simulink model "TD"  (R2020a)
settings: Solver=VariableStepAuto  StartTime=0.0  StopTime=0.05  RelTol=1e-3
undefined symbols (not defined in the file or in its folder): R1, R2
libraries: powerlib x7
settings Model: Creator=eduh_  LastModifiedBy=eduh_

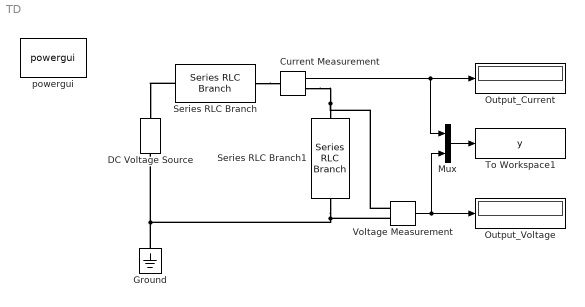
== system TD ==
  Current Measurement : powerlib/Measurements/Current Measurement  PhasorSimulation=off  OutputType=Complex  PSBequivalent=0
  DC Voltage Source : powerlib/Electrical Sources/DC Voltage Source  Amplitude=20  Measurements=None
  Ground : powerlib/Elements/Ground  LConnTagsString=a
  Mux : Mux  Inputs=2
  Output_Current : Display
      settings: Decimation=5
  Output_Voltage : Display
      settings: Decimation=5
  Series RLC Branch : powerlib/Elements/Series RLC Branch  LConnTagsString=__new0  RConnTagsString=__new0  BranchType=R  Resistance=R1  Inductance=0  SetiL0=off  InitialCurrent=0  Capacitance=0  Setx0=off  InitialVoltage=0  Measurements=None
  Series RLC Branch1 : powerlib/Elements/Series RLC Branch  LConnTagsString=__new0  RConnTagsString=__new0  BranchType=R  Resistance=R2  Inductance=0  SetiL0=off  InitialCurrent=0  Capacitance=0  Setx0=off  InitialVoltage=0  Measurements=None
  To Workspace1 : ToWorkspace  VariableName=y  SampleTime=1
      settings: MaxDataPoints=1  Save2DSignal=2-D array (concatenate along first dimension)
  Voltage Measurement : powerlib/Measurements/Voltage Measurement  PhasorSimulation=off  OutputType=Complex  PSBequivalent=0
  powergui : powerlib/powergui  Priority=1  SimulationMode=Discrete  SampleTime=5e-7  frequency=60  Iterations=50  frequencyindice=0  Pbase=100e6  ErrMax=1e-4  UnitsV=kV  UnitsW=MW  buscounter=0  FunctionMessages=off  echomessages=off  EnableUseOfTLC=off  CurrentSourceSwitches=off  DisableSnubberDevices=off  DisableRonSwitches=off  DisableVfSwitches=off  DisplayEquations=off  AutomaticDiscreteSolvers=off  SolverType=Tustin/Backward Euler (TBE)  Interpol=off  ExternalGateDelay=off  methode=off  Ts=100  x0status=blocks  SPID=off  SwTol=0  HookPort=off  NonlinearTolerance=1e-4  nMaxIteration=100  ContinueOnMaxIteration=off  RestoreLinks=warning  ResistiveCurrentMeasurement=off  Frange=[0:2:500]  Ylog=off  Xlog=on  ShowGrid=off  save=off  variable=ZData  structure=0  ZoomFFT=off  StartTime=0.0  cycles=1  DisplayStyle=1  fundamental=60  FreqAxis=off  MaxFrequency=1000  frequencyindicesteady=1  RmsSteady=1  display=off
  wires:
  Voltage Measurement/1 -> Mux/2, Output_Voltage/1
  Current Measurement/1 -> Mux/1, Output_Current/1
  Mux/1 -> To Workspace1/1
  connections:
  Voltage Measurement/LConn1 -- Current Measurement/RConn1 -- Series RLC Branch1/LConn1
  Series RLC Branch1/RConn1 -- Ground/LConn1 -- DC Voltage Source/LConn1 -- Voltage Measurement/LConn2
  Series RLC Branch/LConn1 -- DC Voltage Source/RConn1
  Series RLC Branch/RConn1 -- Current Measurement/LConn1
